simulink library "NFSModelsLibrary"  (R2020a)
settings: Solver=VariableStepAuto  StartTime=0.0  StopTime=10.0  RelTol=1e-3
undefined symbols (not defined in the file or in its folder): Earth, F, Light, MIL, Newton, nfs, Raphson, sigbuilder_block, WGS84
libraries: sharedutil x3, simulink x2, ModelsLibrary x2, $bdroot x2, aerolibwind2 x2, aerolibtransform2 x1
(part 3 of 3)

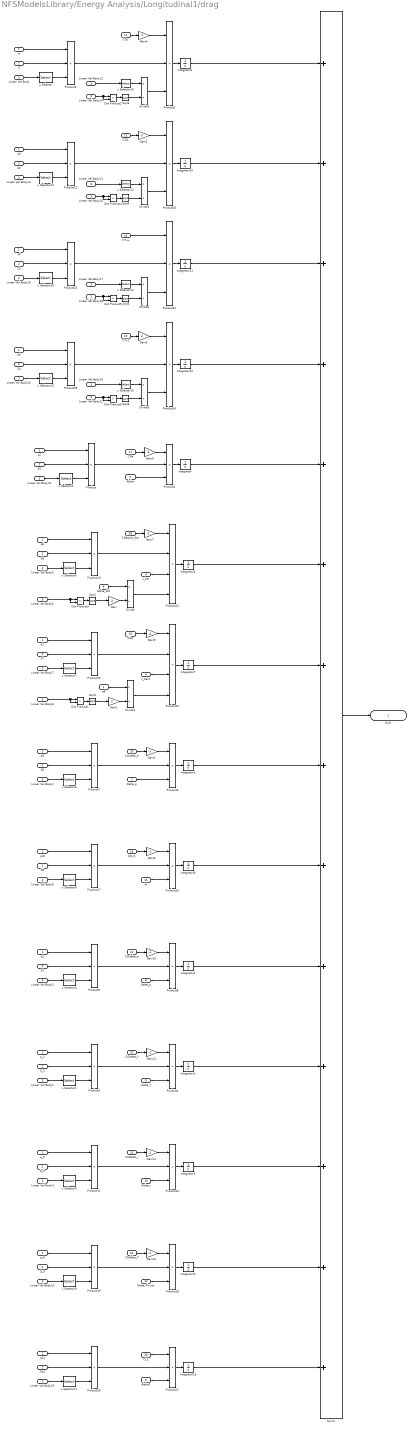
== system NFSModelsLibrary/Energy Analysis/Longitudinal1/drag ==
  q : Inport
  S : Inport  Port=2
  Linear Vel Body : Inport  Port=3
  c_bar : Inport  Port=4
  Alpha : Inport  Port=5
  Alpha_dot : Inport  Port=6
  Delta_e : Inport  Port=7
  Delta_a : Inport  Port=8
  Delta_f : Inport  Port=9
  Delta_r : Inport  Port=10
  iH : Inport  Port=11
  Delta_Thrust : Inport  Port=12
  CD1 : Inport  Port=13
  CDu : Inport  Port=14
  CTx1 : Inport  Port=15
  CTxu : Inport  Port=16
  CDa : Inport  Port=17
  CDalpha_dot : Inport  Port=18
  CDq : Inport  Port=19
  CDdelta_e : Inport  Port=20
  CDdelta_a : Inport  Port=21
  CDdelta_f : Inport  Port=22
  CDdelta_r : Inport  Port=23
  CDdelta_T : Inport  Port=24
  CD_ih : Inport  Port=25
  CL1 : Inport  Port=26
  Alpha1 : InportShadow  Port=5
  Divide{,1..5} (6 alike) : Product  Inputs=*/
  Dot Product{1..6} (6 alike) : DotProduct  InputSameDT=on  OutDataTypeStr=Inherit: Inherit via internal rule
  Gain : Gain  Gain=2
  Gain1 : Gain  Gain=2
  Gain{4..13} (10 alike) : Gain  Gain=-1
  Gain2 : Gain  Gain=-2
  Gain3 : Gain  Gain=2
  Integrator{,1..13} (14 alike) : Integrator
  Linear Vel Body{1..23} (23 alike) : InportShadow  Port=3
  Product{,1..11,13,15..27} (26 alike) : Product  Inputs=3
  Product12 : Product  Inputs=4
  Product14 : Product  Inputs=4
  S{1..10} (10 alike) : InportShadow  Port=2
  S_2 : InportShadow  Port=2
  S_5 : InportShadow  Port=2
  S_9 : InportShadow  Port=2
  Sqrt{1..6} (6 alike) : Sqrt  SaturateOnIntegerOverflow=on
  Sum3 : Sum  Inputs=++++++++++++++
  c_bar1 : InportShadow  Port=4
  q{1..11} (11 alike) : InportShadow
  q_2 : InportShadow
  q_5 : InportShadow
  q_9 : InportShadow
  u Selector{,1..17} (18 alike) : Selector  InputPortWidth=3  IndexOptions=Index vector (dialog)  Indices=[1]  OutputSizes=1
  Out1 : Outport  VectorParamsAs1DForOutWhenUnconnected=off
  wires:
  Integrator1/1 -> Sum3/1
  CDu/1 -> Gain4/1
  Product3/1 -> Product2/2
  Divide2/1 -> Product2/3
  Product2/1 -> Integrator1/1
  Integrator10/1 -> Sum3/2
  q/1 -> Product3/1
  S/1 -> Product3/2
  Sum3/1 -> Out1/1
  u Selector/1 -> Product3/3
  Linear Vel Body/1 -> u Selector/1
  Sqrt3/1 -> Divide2/2
  u Selector10/1 -> Divide2/1
  Dot Product2/1 -> Sqrt3/1
  Linear Vel Body14/1 -> Dot Product2/1, Dot Product2/2
  Linear Vel Body12/1 -> u Selector10/1
  Integrator6/1 -> Sum3/6
  Integrator3/1 -> Sum3/8
  Integrator4/1 -> Sum3/10
  Integrator2/1 -> Sum3/11
  Integrator5/1 -> Sum3/12
  CDdelta_T/1 -> Gain13/1
  Product19/1 -> Product18/2
  Delta_Thrust/1 -> Product18/3
  Product18/1 -> Integrator9/1
  q_9/1 -> Product19/1
  S_9/1 -> Product19/2
  u Selector9/1 -> Product19/3
  Linear Vel Body10/1 -> u Selector9/1
  Integrator9/1 -> Sum3/13
  CDdelta_r/1 -> Gain11/1
  Product11/1 -> Product10/2
  Delta_r/1 -> Product10/3
  Product10/1 -> Integrator5/1
  q_5/1 -> Product11/1
  S_5/1 -> Product11/2
  u Selector5/1 -> Product11/3
  Linear Vel Body4/1 -> u Selector5/1
  CDdelta_f/1 -> Gain12/1
  Product5/1 -> Product4/2
  Delta_f/1 -> Product4/3
  Product4/1 -> Integrator2/1
  q_2/1 -> Product5/1
  S_2/1 -> Product5/2
  u Selector1/1 -> Product5/3
  Linear Vel Body1/1 -> u Selector1/1
  Alpha/1 -> Product1/3
  CDa/1 -> Gain5/1
  Product/1 -> Product1/2
  Product1/1 -> Integrator/1
  q2/1 -> Product/1
  S5/1 -> Product/2
  Linear Vel Body22/1 -> u Selector2/1
  u Selector2/1 -> Product/3
  CDdelta_e/1 -> Gain6/1
  Product7/1 -> Product6/2
  Delta_e/1 -> Product6/3
  Product6/1 -> Integrator3/1
  q9/1 -> Product7/1
  S8/1 -> Product7/2
  u Selector3/1 -> Product7/3
  Linear Vel Body2/1 -> u Selector3/1
  CDdelta_a/1 -> Gain10/1
  Product9/1 -> Product8/2
  Delta_a/1 -> Product8/3
  Product8/1 -> Integrator4/1
  q1/1 -> Product9/1
  S1/1 -> Product9/2
  u Selector4/1 -> Product9/3
  Linear Vel Body3/1 -> u Selector4/1
  CDalpha_dot/1 -> Gain7/1
  Product13/1 -> Product12/2
  c_bar/1 -> Product12/3
  Product12/1 -> Integrator6/1
  q6/1 -> Product13/1
  S6/1 -> Product13/2
  u Selector6/1 -> Product13/3
  Linear Vel Body5/1 -> u Selector6/1
  Gain/1 -> Divide/2
  Alpha_dot/1 -> Divide/1
  Divide/1 -> Product12/4
  Dot Product3/1 -> Sqrt1/1
  Linear Vel Body6/1 -> Dot Product3/1, Dot Product3/2
  Sqrt1/1 -> Gain/1
  CDq/1 -> Gain9/1
  Product15/1 -> Product14/2
  c_bar1/1 -> Product14/3
  Product14/1 -> Integrator7/1
  q7/1 -> Product15/1
  S7/1 -> Product15/2
  u Selector7/1 -> Product15/3
  Linear Vel Body7/1 -> u Selector7/1
  Gain1/1 -> Divide1/2
  q8/1 -> Divide1/1
  Divide1/1 -> Product14/4
  Dot Product1/1 -> Sqrt2/1
  Linear Vel Body8/1 -> Dot Product1/2, Dot Product1/1
  Sqrt2/1 -> Gain1/1
  CD_ih/1 -> Gain8/1
  Product17/1 -> Product16/2
  iH/1 -> Product16/3
  Product16/1 -> Integrator8/1
  q10/1 -> Product17/1
  S9/1 -> Product17/2
  u Selector8/1 -> Product17/3
  Linear Vel Body9/1 -> u Selector8/1
  Integrator8/1 -> Sum3/9
  Integrator/1 -> Sum3/5
  CD1/1 -> Gain2/1
  Product21/1 -> Product20/2
  Divide3/1 -> Product20/3
  Product20/1 -> Integrator10/1
  q3/1 -> Product21/1
  S2/1 -> Product21/2
  u Selector11/1 -> Product21/3
  Linear Vel Body13/1 -> u Selector11/1
  Sqrt4/1 -> Divide3/2
  u Selector12/1 -> Divide3/1
  Dot Product4/1 -> Sqrt4/1
  Linear Vel Body15/1 -> Dot Product4/2, Dot Product4/1
  Linear Vel Body11/1 -> u Selector12/1
  Gain2/1 -> Product20/1
  CTxu/1 -> Product22/1
  Product23/1 -> Product22/2
  Divide4/1 -> Product22/3
  Product22/1 -> Integrator11/1
  q4/1 -> Product23/1
  S3/1 -> Product23/2
  u Selector13/1 -> Product23/3
  Linear Vel Body16/1 -> u Selector13/1
  Sqrt5/1 -> Divide4/2
  u Selector14/1 -> Divide4/1
  Dot Product5/1 -> Sqrt5/1
  Linear Vel Body18/1 -> Dot Product5/1, Dot Product5/2
  Linear Vel Body17/1 -> u Selector14/1
  Integrator11/1 -> Sum3/3
  CTx1/1 -> Gain3/1
  Product25/1 -> Product24/2
  Divide5/1 -> Product24/3
  Product24/1 -> Integrator12/1
  q5/1 -> Product25/1
  S4/1 -> Product25/2
  u Selector15/1 -> Product25/3
  Linear Vel Body20/1 -> u Selector15/1
  Sqrt6/1 -> Divide5/2
  u Selector16/1 -> Divide5/1
  Dot Product6/1 -> Sqrt6/1
  Linear Vel Body21/1 -> Dot Product6/2, Dot Product6/1
  Linear Vel Body19/1 -> u Selector16/1
  Gain3/1 -> Product24/1
  Integrator12/1 -> Sum3/4
  Integrator7/1 -> Sum3/7
  Alpha1/1 -> Product27/3
  CL1/1 -> Product27/1
  Product26/1 -> Product27/2
  Product27/1 -> Integrator13/1
  q11/1 -> Product26/1
  S10/1 -> Product26/2
  Linear Vel Body23/1 -> u Selector17/1
  u Selector17/1 -> Product26/3
  Integrator13/1 -> Sum3/14
  Gain4/1 -> Product2/1
  Gain5/1 -> Product1/1
  Gain6/1 -> Product6/1
  Gain7/1 -> Product12/1
  Gain9/1 -> Product14/1
  Gain8/1 -> Product16/1
  Gain10/1 -> Product8/1
  Gain12/1 -> Product4/1
  Gain11/1 -> Product10/1
  Gain13/1 -> Product18/1

== system NFSModelsLibrary/Forces and Moments/Thrust/Signal Builder ==
  Demux : Demux  Tag=STV Demux  Outputs=1
      settings: DisplayOption=none
  FromWs : FromWorkspace  Tag=STV FromWs  VariableName=tuvar
      SigBuilderData=|
      | common.afterFinalStr = 'Extrapolate'
      | common.sampleTime = 0
      | dataSet.timeRange = [0 1200]
      | dataSet.name = 'Thrust Deviation'
      | sbobj.Groups.Name = 'Thrust Deviation'
      | sbobj.Groups.Signals.Name = 'ThrustDeviation'
      | sbobj.Groups.Signals.XData = [0 10 10 12 12 1200]
      | sbobj.Groups.Signals.YData = [1 1 1.05 1.05 1 1]
      | sbobj.Groups.TimeRange = [0 1200]
  ThrustDeviation : Outport  Tag=STV Outport  VectorParamsAs1DForOutWhenUnconnected=off
  wires:
  Demux/1 -> ThrustDeviation/1
  FromWs/1 -> Demux/1

== system NFSModelsLibrary/Forces and Moments/Weight/Vector Magnitude ==
  Vector : Inport
  Dot Product : DotProduct  InputSameDT=on  OutDataTypeStr=Inherit: Inherit via internal rule
  Sqrt : Sqrt  SaturateOnIntegerOverflow=on
  Vector Magnitude : Outport  VectorParamsAs1DForOutWhenUnconnected=off
  wires:
  Sqrt/1 -> Vector Magnitude/1  "abs(V)"
  Vector/1 -> Dot Product/2, Dot Product/1
  Dot Product/1 -> Sqrt/1

== system NFSModelsLibrary/Aerodynamic Forces and Moments Derivatives/Forces/Aerodynamic Forces/Wind2Body TM ==
  Alpha : Inport  PortDimensions=1
  Beta : Inport  Port=2  PortDimensions=1
  ChSign : Gain  Gain=-1  SaturateOnIntegerOverflow=on  OutDataTypeStr=Inherit: Same as input  ParamDataTypeStr=Inherit: Same as input
  ChSign1 : Gain  Gain=-1  SaturateOnIntegerOverflow=on  OutDataTypeStr=Inherit: Same as input  ParamDataTypeStr=Inherit: Same as input
  ChSign2 : Gain  Gain=-1  SaturateOnIntegerOverflow=on  OutDataTypeStr=Inherit: Same as input  ParamDataTypeStr=Inherit: Same as input
  Product{,1..3} (4 alike) : Product  InputSameDT=on  SaturateOnIntegerOverflow=on  OutDataTypeStr=Inherit: Same as first input
  S Matrix : Concatenate  NumInputs=3  Mode=Multidimensional array  ConcatenateDimension=2
  S Col1 : Concatenate  NumInputs=3  Mode=Multidimensional array
  S Col2 : Concatenate  NumInputs=3  Mode=Multidimensional array
  S Col3 : Concatenate  NumInputs=3  Mode=Multidimensional array
  Trigonometric Function : Trigonometry
  Trigonometric Function1 : Trigonometry  Operator=cos
  Trigonometric Function2 : Trigonometry
  Trigonometric Function3 : Trigonometry  Operator=cos
  Zero : Constant  Value=0
  T_BW : Outport  PortDimensions=[3,3]  VectorParamsAs1DForOutWhenUnconnected=off
  wires:
  Alpha/1 -> Trigonometric Function/1, Trigonometric Function1/1
  Beta/1 -> Trigonometric Function3/1, Trigonometric Function2/1
  Trigonometric Function/1 -> ChSign1/1, Product2/1, Product3/1
  Trigonometric Function1/1 -> Product1/1, S Col3/3, Product/1
  Trigonometric Function2/1 -> Product1/2, S Col2/1, Product3/2
  Trigonometric Function3/1 -> Product/2, S Col2/2, Product2/2
  Product1/1 -> ChSign/1
  Product/1 -> S Col1/1
  ChSign/1 -> S Col1/2
  ChSign1/1 -> S Col1/3
  Zero/1 -> S Col2/3
  Product3/1 -> ChSign2/1
  Product2/1 -> S Col3/1
  ChSign2/1 -> S Col3/2
  S Col1/1 -> S Matrix/1
  S Col2/1 -> S Matrix/2
  S Col3/1 -> S Matrix/3
  S Matrix/1 -> T_BW/1

== system NFSModelsLibrary/Aerodynamic Forces and Moments Derivatives/Forces/Force Coefficients Calculator/Drag Coefficient ==
  CL : Inport  PortDimensions=1
  alpha : Inport  Port=2  PortDimensions=1
  DeltaElevator : Inport  Port=3  PortDimensions=1
  DeltaFlap : Inport  Port=4  PortDimensions=1
  DeltaAileron : Inport  Port=5  PortDimensions=1
  DeltaRudder : Inport  Port=6  PortDimensions=1
  Mach : Inport  Port=7  PortDimensions=1
  Abs{,1..4} (5 alike) : Abs  SaturateOnIntegerOverflow=on
  CD0 : Constant  Value=cD0
  CL^2 : Math  Operator=square  SignedPower=on  SaturateOnIntegerOverflow=on
  Induced Drag : Gain  Gain=nfs.aero.k  SaturateOnIntegerOverflow=on  OutDataTypeStr=Inherit: Same as input  ParamDataTypeStr=Inherit: Same as input
  Sum2 : Sum  Inputs=++++++++  InputSameDT=on  SaturateOnIntegerOverflow=on  OutDataTypeStr=Inherit: Same as first input
  cDM : Gain  Gain=nfs.aero.cDM  SaturateOnIntegerOverflow=on  OutDataTypeStr=Inherit: Same as input  ParamDataTypeStr=Inherit: Same as input
  cDalpha : Gain  Gain=nfs.aero.cDalpha  SaturateOnIntegerOverflow=on  OutDataTypeStr=Inherit: Same as input  ParamDataTypeStr=Inherit: Same as input
  cDdelta_a : Gain  Gain=nfs.aero.cDdelta_a  SaturateOnIntegerOverflow=on  OutDataTypeStr=Inherit: Same as input  ParamDataTypeStr=Inherit: Same as input
  cDdelta_e : Gain  Gain=nfs.aero.cDdelta_e  SaturateOnIntegerOverflow=on  OutDataTypeStr=Inherit: Same as input  ParamDataTypeStr=Inherit: Same as input
  cDdelta_f : Gain  Gain=nfs.aero.cDdelta_f  SaturateOnIntegerOverflow=on  OutDataTypeStr=Inherit: Same as input  ParamDataTypeStr=Inherit: Same as input
  cDdelta_r : Gain  Gain=nfs.aero.cDdelta_r  SaturateOnIntegerOverflow=on  OutDataTypeStr=Inherit: Same as input  ParamDataTypeStr=Inherit: Same as input
  CD : Outport  PortDimensions=1  VectorParamsAs1DForOutWhenUnconnected=off
  wires:
  Abs4/1 -> Sum2/3
  cDM/1 -> Sum2/8
  Abs3/1 -> Sum2/7
  Abs2/1 -> Sum2/6
  Abs1/1 -> Sum2/5
  Abs/1 -> Sum2/4
  cDalpha/1 -> Abs4/1
  alpha/1 -> cDalpha/1
  CL^2/1 -> Induced Drag/1
  CD0/1 -> Sum2/1
  Induced Drag/1 -> Sum2/2
  cDdelta_f/1 -> Abs/1
  cDdelta_e/1 -> Abs1/1
  cDdelta_a/1 -> Abs2/1
  cDdelta_r/1 -> Abs3/1
  CL/1 -> CL^2/1
  Mach/1 -> cDM/1
  DeltaFlap/1 -> cDdelta_f/1
  DeltaElevator/1 -> cDdelta_e/1
  DeltaAileron/1 -> cDdelta_a/1
  DeltaRudder/1 -> cDdelta_r/1
  Sum2/1 -> CD/1

== system NFSModelsLibrary/Aerodynamic Forces and Moments Derivatives/Forces/Force Coefficients Calculator/Lift Coefficient ==
  Linear Velocity : Inport  PortDimensions=[3 1]
  Alpha : Inport  Port=2  PortDimensions=1
  DeltaElevator : Inport  Port=3  PortDimensions=1
  DeltaFlap : Inport  Port=4  PortDimensions=1
  Alphadot : Inport  Port=5  PortDimensions=1
  Q : Inport  Port=6  PortDimensions=1
  Mach : Inport  Port=7  PortDimensions=1
  1 : Gain  Gain=2  SaturateOnIntegerOverflow=on  OutDataTypeStr=Inherit: Same as input  ParamDataTypeStr=Inherit: Same as input
  CL*c/(2V) : Product  Inputs=**/  InputSameDT=on  SaturateOnIntegerOverflow=on  OutDataTypeStr=Inherit: Same as first input
  CL0 : Constant  Value=cL0
  CLM : Gain  Gain=nfs.aero.cLM  SaturateOnIntegerOverflow=on  OutDataTypeStr=Inherit: Same as input  ParamDataTypeStr=Inherit: Same as input
  Sum1 : Sum  InputSameDT=on  SaturateOnIntegerOverflow=on  OutDataTypeStr=Inherit: Same as first input
  Sum3 : Sum  Inputs=++++++  InputSameDT=on  SaturateOnIntegerOverflow=on  OutDataTypeStr=Inherit: Same as first input
  Velocity Magnitude : Subsystem
  Wing chord1 : Constant  Value=meanchord
  cLalpha : Gain  Gain=nfs.aero.cLalpha  SaturateOnIntegerOverflow=on  OutDataTypeStr=Inherit: Same as input  ParamDataTypeStr=Inherit: Same as input
  cLalphadot : Gain  Gain=nfs.aero.cLalphadot  SaturateOnIntegerOverflow=on  OutDataTypeStr=Inherit: Same as input  ParamDataTypeStr=Inherit: Same as input
  cLdelta_e : Gain  Gain=nfs.aero.cLdelta_e  SaturateOnIntegerOverflow=on  OutDataTypeStr=Inherit: Same as input  ParamDataTypeStr=Inherit: Same as input
  cLdelta_f : Gain  Gain=nfs.aero.cLdelta_f  SaturateOnIntegerOverflow=on  OutDataTypeStr=Inherit: Same as input  ParamDataTypeStr=Inherit: Same as input
  cLq : Gain  Gain=nfs.aero.cLq  SaturateOnIntegerOverflow=on  OutDataTypeStr=Inherit: Same as input  ParamDataTypeStr=Inherit: Same as input
  CL : Outport  PortDimensions=1  VectorParamsAs1DForOutWhenUnconnected=off
  wires:
  CLM/1 -> Sum3/6
  1/1 -> CL*c/(2V)/3
  Wing chord1/1 -> CL*c/(2V)/2
  cLq/1 -> Sum1/2
  Alpha/1 -> cLalpha/1
  DeltaElevator/1 -> cLdelta_e/1
  DeltaFlap/1 -> cLdelta_f/1
  cLalphadot/1 -> Sum1/1
  Sum1/1 -> CL*c/(2V)/1
  CL0/1 -> Sum3/1
  cLalpha/1 -> Sum3/2
  cLdelta_e/1 -> Sum3/3
  cLdelta_f/1 -> Sum3/4
  CL*c/(2V)/1 -> Sum3/5
  Mach/1 -> CLM/1
  Linear Velocity/1 -> Velocity Magnitude/1(Velocity)
  Velocity Magnitude/1(Velocity Magnitude) -> 1/1
  Alphadot/1 -> cLalphadot/1
  Q/1 -> cLq/1
  Sum3/1 -> CL/1

== system NFSModelsLibrary/Aerodynamic Forces and Moments Derivatives/Forces/Force Coefficients Calculator/SideForce Coefficient ==
  Linear Velocity : Inport  PortDimensions=[3 1]
  Beta : Inport  Port=2  PortDimensions=1
  P : Inport  Port=3  PortDimensions=1
  R : Inport  Port=4  PortDimensions=1
  DeltaAileron : Inport  Port=5  PortDimensions=1
  DeltaRudder : Inport  Port=6  PortDimensions=1
  2 : Gain  Gain=2  SaturateOnIntegerOverflow=on  OutDataTypeStr=Inherit: Same as input  ParamDataTypeStr=Inherit: Same as input
  CY*b/(2V) : Product  Inputs=**/  InputSameDT=on  SaturateOnIntegerOverflow=on  OutDataTypeStr=Inherit: Same as first input
  Sum : Sum  InputSameDT=on  SaturateOnIntegerOverflow=on  OutDataTypeStr=Inherit: Same as first input
  Sum2 : Sum  Inputs=++++  InputSameDT=on  SaturateOnIntegerOverflow=on  OutDataTypeStr=Inherit: Same as first input
  Velocity Magnitude : Subsystem
  Wing span : Constant  Value=nfs.span
  cYbeta : Gain  Gain=nfs.aero.cYbeta  SaturateOnIntegerOverflow=on  OutDataTypeStr=Inherit: Same as input  ParamDataTypeStr=Inherit: Same as input
  cYdelta_a : Gain  Gain=nfs.aero.cYdelta_a  SaturateOnIntegerOverflow=on  OutDataTypeStr=Inherit: Same as input  ParamDataTypeStr=Inherit: Same as input
  cYdelta_r : Gain  Gain=nfs.aero.cYdelta_r  SaturateOnIntegerOverflow=on  OutDataTypeStr=Inherit: Same as input  ParamDataTypeStr=Inherit: Same as input
  cYp : Gain  Gain=nfs.aero.cYp  SaturateOnIntegerOverflow=on  OutDataTypeStr=Inherit: Same as input  ParamDataTypeStr=Inherit: Same as input
  cYr : Gain  Gain=nfs.aero.cYr  SaturateOnIntegerOverflow=on  OutDataTypeStr=Inherit: Same as input  ParamDataTypeStr=Inherit: Same as input
  CY : Outport  VectorParamsAs1DForOutWhenUnconnected=off
  wires:
  cYp/1 -> Sum/1
  cYr/1 -> Sum/2
  Sum/1 -> CY*b/(2V)/1
  Wing span/1 -> CY*b/(2V)/2
  2/1 -> CY*b/(2V)/3
  cYbeta/1 -> Sum2/1
  cYdelta_a/1 -> Sum2/2
  cYdelta_r/1 -> Sum2/3
  CY*b/(2V)/1 -> Sum2/4
  Beta/1 -> cYbeta/1
  Linear Velocity/1 -> Velocity Magnitude/1(Velocity)
  Velocity Magnitude/1(Velocity Magnitude) -> 2/1
  DeltaAileron/1 -> cYdelta_a/1
  DeltaRudder/1 -> cYdelta_r/1
  P/1 -> cYp/1
  R/1 -> cYr/1
  Sum2/1 -> CY/1

== system NFSModelsLibrary/Aerodynamic Forces and Moments Derivatives/Moments/Aerodynamic Moment /Wind2Body TM ==
  Alpha : Inport  PortDimensions=1
  Beta : Inport  Port=2  PortDimensions=1
  ChSign : Gain  Gain=-1  SaturateOnIntegerOverflow=on  OutDataTypeStr=Inherit: Same as input  ParamDataTypeStr=Inherit: Same as input
  ChSign1 : Gain  Gain=-1  SaturateOnIntegerOverflow=on  OutDataTypeStr=Inherit: Same as input  ParamDataTypeStr=Inherit: Same as input
  ChSign2 : Gain  Gain=-1  SaturateOnIntegerOverflow=on  OutDataTypeStr=Inherit: Same as input  ParamDataTypeStr=Inherit: Same as input
  Product{,1..3} (4 alike) : Product  InputSameDT=on  SaturateOnIntegerOverflow=on  OutDataTypeStr=Inherit: Same as first input
  S Matrix : Concatenate  NumInputs=3  Mode=Multidimensional array  ConcatenateDimension=2
  S Col1 : Concatenate  NumInputs=3  Mode=Multidimensional array
  S Col2 : Concatenate  NumInputs=3  Mode=Multidimensional array
  S Col3 : Concatenate  NumInputs=3  Mode=Multidimensional array
  Trigonometric Function : Trigonometry
  Trigonometric Function1 : Trigonometry  Operator=cos
  Trigonometric Function2 : Trigonometry
  Trigonometric Function3 : Trigonometry  Operator=cos
  Zero : Constant  Value=0
  T_BW : Outport  PortDimensions=[3,3]  VectorParamsAs1DForOutWhenUnconnected=off
  wires:
  Alpha/1 -> Trigonometric Function/1, Trigonometric Function1/1
  Beta/1 -> Trigonometric Function3/1, Trigonometric Function2/1
  Trigonometric Function/1 -> ChSign1/1, Product2/1, Product3/1
  Trigonometric Function1/1 -> Product1/1, S Col3/3, Product/1
  Trigonometric Function2/1 -> Product1/2, S Col2/1, Product3/2
  Trigonometric Function3/1 -> Product/2, S Col2/2, Product2/2
  Product1/1 -> ChSign/1
  Product/1 -> S Col1/1
  ChSign/1 -> S Col1/2
  ChSign1/1 -> S Col1/3
  Zero/1 -> S Col2/3
  Product3/1 -> ChSign2/1
  Product2/1 -> S Col3/1
  ChSign2/1 -> S Col3/2
  S Col1/1 -> S Matrix/1
  S Col2/1 -> S Matrix/2
  S Col3/1 -> S Matrix/3
  S Matrix/1 -> T_BW/1

== system NFSModelsLibrary/Aerodynamic Forces and Moments Derivatives/Moments/Pitch Moment Coefficient/Velocity Magnitude ==
  Velocity : Inport
  Dot Product : DotProduct  InputSameDT=on  OutDataTypeStr=Inherit: Inherit via internal rule
  Sqrt : Sqrt  SaturateOnIntegerOverflow=on
  Velocity Magnitude : Outport  VectorParamsAs1DForOutWhenUnconnected=off
  wires:
  Dot Product/1 -> Sqrt/1
  Velocity/1 -> Dot Product/1, Dot Product/2
  Sqrt/1 -> Velocity Magnitude/1  "abs(V)"

== system NFSModelsLibrary/Aerodynamic Forces and Moments Derivatives/Moments/Roll Moment Coefficient/Velocity Magnitude ==
  Velocity : Inport
  Dot Product : DotProduct  InputSameDT=on  OutDataTypeStr=Inherit: Inherit via internal rule
  Sqrt : Sqrt  SaturateOnIntegerOverflow=on
  Velocity Magnitude : Outport  VectorParamsAs1DForOutWhenUnconnected=off
  wires:
  Dot Product/1 -> Sqrt/1
  Velocity/1 -> Dot Product/1, Dot Product/2
  Sqrt/1 -> Velocity Magnitude/1  "abs(V)"

== system NFSModelsLibrary/Aerodynamic Forces and Moments Derivatives/Moments/Yaw Moment Coefficient/Velocity Magnitude ==
  Velocity : Inport
  Dot Product : DotProduct  InputSameDT=on  OutDataTypeStr=Inherit: Inherit via internal rule
  Sqrt : Sqrt  SaturateOnIntegerOverflow=on
  Velocity Magnitude : Outport  VectorParamsAs1DForOutWhenUnconnected=off
  wires:
  Dot Product/1 -> Sqrt/1
  Velocity/1 -> Dot Product/1, Dot Product/2
  Sqrt/1 -> Velocity Magnitude/1  "abs(V)"

== system NFSModelsLibrary/Aerodynamic Forces and Moments Derivatives/Turbulence/Turbulence Model/Dryden Turbulence Model ==
  In : Inport
  Bus Creator2 : BusCreator  Inputs=2
  Bus Selector1 : BusSelector  OutputSignals=Altitude,Linear Velocity,DCM
  Bus Selector2 : BusSelector  OutputSignals=Linear Velocity,Angular Velocity
  Dryden Wind Turbulence Model (Continuous (+q +r)) : aerolibwind2/Dryden Wind Turbulence Model  (Continuous (+q -r))  units=Metric (MKS)  spec=MIL-F-8785C  model=Continuous Dryden (+q +r)  W20=15  Wdeg=0  TurbProb=10^-2 - Light  L_high=nfs.Uncertainty.Turbulence.Dryden.ScaleLength  Wingspan=nfs.span  ts=nfs.Uncertainty.Noise.SampleTime  Seed=nfs.Uncertainty.Turbulence.Dryden.Seed  T_on=on
  Sum1 : Sum  Inputs=++|
  Sum2 : Sum  Inputs=++|
  Velocity Magnitude : Subsystem
  Out : Outport  VectorParamsAs1DForOutWhenUnconnected=off
  wires:
  Sum1/1 -> Bus Creator2/1  "Linear Velocity"
  Sum2/1 -> Bus Creator2/2  "Angular Velocity"
  Bus Selector2/1 -> Sum1/1  "<Linear Velocity>"
  Bus Selector2/2 -> Sum2/1  "<Angular Velocity>"
  Dryden Wind Turbulence Model (Continuous (+q +r))/1 -> Sum1/2
  Bus Selector1/3 -> Dryden Wind Turbulence Model (Continuous (+q +r))/3  "<DCM>"
  Bus Selector1/2 -> Velocity Magnitude/1(Velocity)  "<Linear Velocity>"
  In/1 -> Bus Selector2/1, Bus Selector1/1
  Velocity Magnitude/1(Velocity Magnitude) -> Dryden Wind Turbulence Model (Continuous (+q +r))/2
  Bus Selector1/1 -> Dryden Wind Turbulence Model (Continuous (+q +r))/1  "<Altitude>"
  Bus Creator2/1 -> Out/1
  Dryden Wind Turbulence Model (Continuous (+q +r))/2 -> Sum2/2

== system NFSModelsLibrary/Aerodynamic Forces and Moments Derivatives/Turbulence/Turbulence Model/No Turbulence ==
  In : Inport
  Bus Creator1 : BusCreator  Inputs=2
  Bus Selector : BusSelector  OutputSignals=Linear Velocity,Angular Velocity
  Out : Outport  VectorParamsAs1DForOutWhenUnconnected=off
  wires:
  Bus Selector/1 -> Bus Creator1/1  "<Linear Velocity>"
  Bus Selector/2 -> Bus Creator1/2  "<Angular Velocity>"
  Bus Creator1/1 -> Out/1
  In/1 -> Bus Selector/1

== system NFSModelsLibrary/Aerodynamic Forces and Moments Derivatives/Turbulence/Turbulence Model/Von-Karman Turbulence Model ==
  In : Inport
  Bus Creator2 : BusCreator  Inputs=2
  Bus Selector1 : BusSelector  OutputSignals=Altitude,Linear Velocity,DCM
  Bus Selector2 : BusSelector  OutputSignals=Linear Velocity,Angular Velocity
  Sum1 : Sum  Inputs=++|
  Sum2 : Sum  Inputs=++|
  Velocity Magnitude : Subsystem
  Von Karman Wind Turbulence Model (Continuous (+q +r)) : aerolibwind2/Dryden Wind Turbulence Model  (Continuous (+q -r))  units=Metric (MKS)  spec=MIL-F-8785C  model=Continuous Von Karman (+q +r)  W20=15  Wdeg=0  TurbProb=10^-2 - Light  L_high=nfs.Uncertainty.Turbulence.VonKarman.ScaleLength  Wingspan=nfs.span  ts=nfs.Uncertainty.Noise.SampleTime  Seed=nfs.Uncertainty.Turbulence.VonKarman.Seed  T_on=on
  Out : Outport  VectorParamsAs1DForOutWhenUnconnected=off
  wires:
  Von Karman Wind Turbulence Model (Continuous (+q +r))/2 -> Sum2/2
  Bus Creator2/1 -> Out/1
  Bus Selector1/1 -> Von Karman Wind Turbulence Model (Continuous (+q +r))/1  "<Altitude>"
  Velocity Magnitude/1(Velocity Magnitude) -> Von Karman Wind Turbulence Model (Continuous (+q +r))/2
  In/1 -> Bus Selector1/1, Bus Selector2/1
  Bus Selector1/2 -> Velocity Magnitude/1(Velocity)  "<Linear Velocity>"
  Bus Selector1/3 -> Von Karman Wind Turbulence Model (Continuous (+q +r))/3  "<DCM>"
  Von Karman Wind Turbulence Model (Continuous (+q +r))/1 -> Sum1/2
  Bus Selector2/2 -> Sum2/1  "<Angular Velocity>"
  Bus Selector2/1 -> Sum1/1  "<Linear Velocity>"
  Sum2/1 -> Bus Creator2/2  "Angular Velocity"
  Sum1/1 -> Bus Creator2/1  "Linear Velocity"

== system NFSModelsLibrary/Aerodynamic Forces and Moments Derivatives/Forces/Force Coefficients Calculator/Lift Coefficient/Velocity Magnitude ==
  Velocity : Inport
  Dot Product : DotProduct  InputSameDT=on  OutDataTypeStr=Inherit: Inherit via internal rule
  Sqrt : Sqrt  SaturateOnIntegerOverflow=on
  Velocity Magnitude : Outport  VectorParamsAs1DForOutWhenUnconnected=off
  wires:
  Dot Product/1 -> Sqrt/1
  Velocity/1 -> Dot Product/1, Dot Product/2
  Sqrt/1 -> Velocity Magnitude/1  "abs(V)"

== system NFSModelsLibrary/Aerodynamic Forces and Moments Derivatives/Forces/Force Coefficients Calculator/SideForce Coefficient/Velocity Magnitude ==
  Velocity : Inport
  Dot Product : DotProduct  InputSameDT=on  OutDataTypeStr=Inherit: Inherit via internal rule
  Sqrt : Sqrt  SaturateOnIntegerOverflow=on
  Velocity Magnitude : Outport  VectorParamsAs1DForOutWhenUnconnected=off
  wires:
  Dot Product/1 -> Sqrt/1
  Velocity/1 -> Dot Product/1, Dot Product/2
  Sqrt/1 -> Velocity Magnitude/1  "abs(V)"

== system NFSModelsLibrary/Aerodynamic Forces and Moments Derivatives/Turbulence/Turbulence Model/Dryden Turbulence Model/Velocity Magnitude ==
  Velocity : Inport
  Dot Product : DotProduct  InputSameDT=on  OutDataTypeStr=Inherit: Inherit via internal rule
  Sqrt : Sqrt  SaturateOnIntegerOverflow=on
  Velocity Magnitude : Outport  VectorParamsAs1DForOutWhenUnconnected=off
  wires:
  Dot Product/1 -> Sqrt/1
  Velocity/1 -> Dot Product/1, Dot Product/2
  Sqrt/1 -> Velocity Magnitude/1  "abs(V)"

== system NFSModelsLibrary/Aerodynamic Forces and Moments Derivatives/Turbulence/Turbulence Model/Von-Karman Turbulence Model/Velocity Magnitude ==
  Velocity : Inport
  Dot Product : DotProduct  InputSameDT=on  OutDataTypeStr=Inherit: Inherit via internal rule
  Sqrt : Sqrt  SaturateOnIntegerOverflow=on
  Velocity Magnitude : Outport  VectorParamsAs1DForOutWhenUnconnected=off
  wires:
  Sqrt/1 -> Velocity Magnitude/1  "abs(V)"
  Velocity/1 -> Dot Product/2, Dot Product/1
  Dot Product/1 -> Sqrt/1
